simulink model "Adoptive_Cruse_control"  (R2024a)
settings: Solver=FixedStepAuto  StartTime=0.0  StopTime=10.0  RelTol=1e-3
settings Model: DataDictionary=Adoptive_cruse_control_data.sldd  Creator=kanna  LastModifiedBy=kanna
settings OptimizationCC: DefaultParameterBehavior=Inlined  EnhancedBackFolding=on  PassReuseOutputArgsAs=Individual arguments  ZeroExternalMemoryAtStartup=off  ZeroInternalMemoryAtStartup=off  OptimizeBlockOrder=speed  DifferentSizesBufferReuse=on  OptimizationCustomize=off  EfficientTunableParamExpr=on
settings DebuggingCC: ParameterTunabilityLossMsg=error
settings SFSimCC: MATLABDynamicMemAlloc=off
settings RTWCC: Description=Embedded Coder  SystemTargetFile=ert.tlc  TemplateMakefile=ert_default_tmf
settings CodeAppCC: ForceParamTrailComments=on  IgnoreCustomStorageClasses=off  OperatorAnnotations=on  SimulinkDataObjDesc=on  SFDataObjDesc=on  InsertBlockDesc=on
settings ERTTargetCC: TargetLangStandard=C99 (ISO)  GenerateSampleERTMain=on  InlinedParameterPlacement=NonHierarchical  ERTCustomFileTemplate=example_file_process.tlc

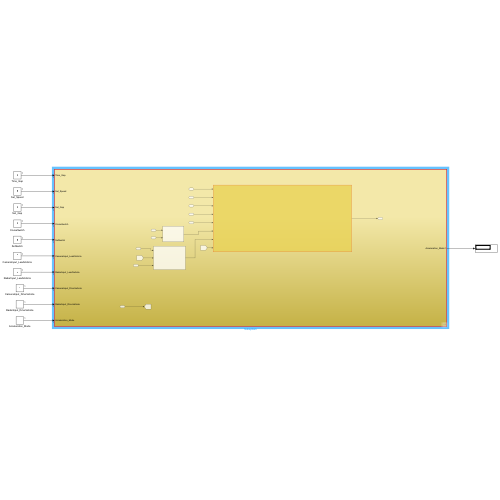
[thumbnail: Simulink's stored preview of the top-level diagram]
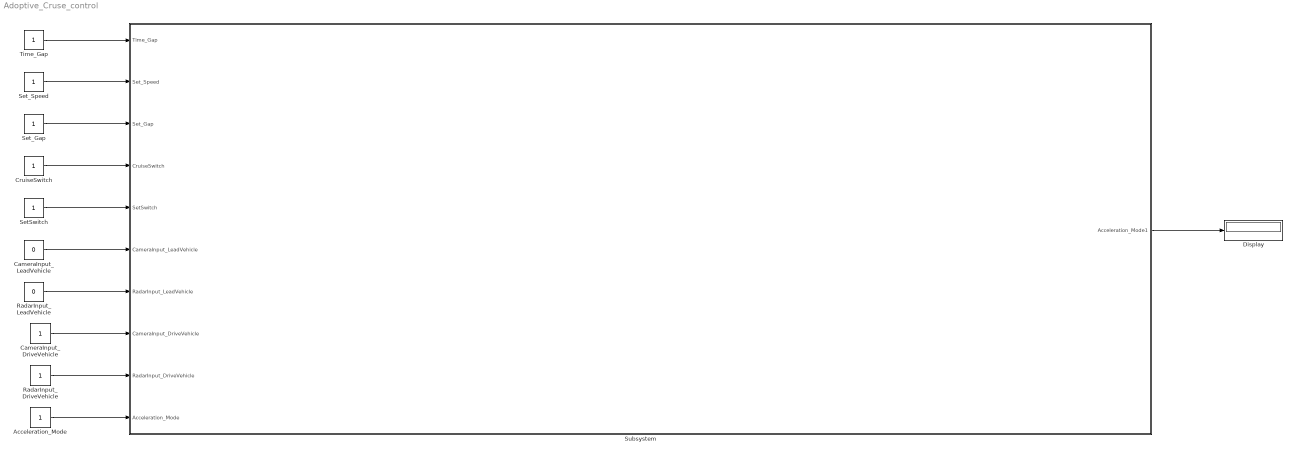
== system Adoptive_Cruse_control ==
  Acceleration_Mode : Constant
  CameraInput_DriveVehicle : Constant
  CameraInput_LeadVehicle : Constant  Value=0
  CruiseSwitch : Constant
  Display : Display
  RadarInput_DriveVehicle : Constant
  RadarInput_LeadVehicle : Constant  Value=0
  SetSwitch : Constant
  Set_Gap : Constant
  Set_Speed : Constant
  Subsystem : Subsystem  TreatAsAtomicUnit=on
  Time_Gap : Constant
  wires:
  Subsystem/1(Acceleration_Mode1) -> Display/1
  Acceleration_Mode/1 -> Subsystem/10(Acceleration_Mode)
  RadarInput_DriveVehicle/1 -> Subsystem/9(RadarInput_DriveVehicle)
  CameraInput_DriveVehicle/1 -> Subsystem/8(CameraInput_DriveVehicle)
  RadarInput_LeadVehicle/1 -> Subsystem/7(RadarInput_LeadVehicle)
  CameraInput_LeadVehicle/1 -> Subsystem/6("CameraInput_LeadVehicle ")
  SetSwitch/1 -> Subsystem/5(SetSwitch)
  CruiseSwitch/1 -> Subsystem/4(CruiseSwitch)
  Set_Gap/1 -> Subsystem/3(Set_Gap)
  Set_Speed/1 -> Subsystem/2(Set_Speed)
  Time_Gap/1 -> Subsystem/1(Time_Gap)

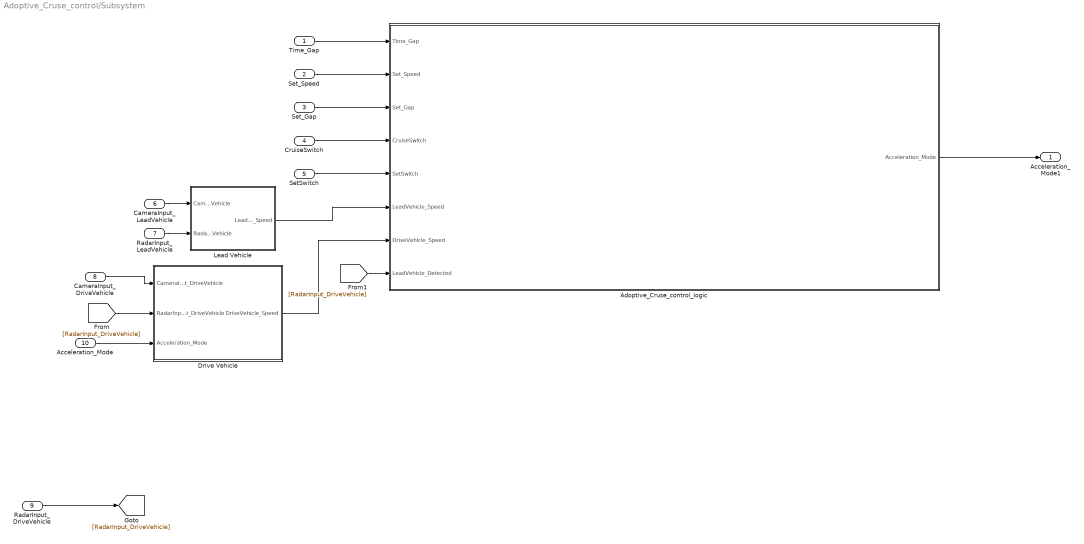
== system Adoptive_Cruse_control/Subsystem ==
  Time_Gap : Inport
  Set_Speed : Inport  Port=2
  Set_Gap : Inport  Port=3
  CruiseSwitch : Inport  Port=4
  SetSwitch : Inport  Port=5
  "CameraInput_LeadVehicle " : Inport  Port=6
  RadarInput_LeadVehicle : Inport  Port=7
  CameraInput_DriveVehicle : Inport  Port=8
  RadarInput_DriveVehicle : Inport  Port=9
  Acceleration_Mode : Inport  Port=10
  Adoptive_Cruse_control_logic : Subsystem
  Drive Vehicle : Subsystem
  Lead Vehicle : Subsystem
  Acceleration_Mode1 : Outport
  wires:
  Drive Vehicle/1("DriveVehicle_Speed ") -> Adoptive_Cruse_control_logic/7("DriveVehicle_Speed ")
  Acceleration_Mode/1 -> Drive Vehicle/3(Acceleration_Mode)
  RadarInput_LeadVehicle/1 -> Lead Vehicle/2(RadarInput_LeadVehicle)
  Set_Gap/1 -> Adoptive_Cruse_control_logic/3(Set_Gap)
  CameraInput_DriveVehicle/1 -> Drive Vehicle/1(CameraInput_DriveVehicle)
  CruiseSwitch/1 -> Adoptive_Cruse_control_logic/4(CruiseSwitch)
  Set_Speed/1 -> Adoptive_Cruse_control_logic/2(Set_Speed)
  Lead Vehicle/1(LeadVehicle_Speed) -> Adoptive_Cruse_control_logic/6(LeadVehicle_Speed)
  "CameraInput_LeadVehicle "/1 -> Lead Vehicle/1("CameraInput_LeadVehicle ")
  SetSwitch/1 -> Adoptive_Cruse_control_logic/5(SetSwitch)
  Time_Gap/1 -> Adoptive_Cruse_control_logic/1(Time_Gap)
  Adoptive_Cruse_control_logic/1(Acceleration_Mode) -> Acceleration_Mode1/1
  RadarInput_DriveVehicle/1 -> [RadarInput_DriveVehicle]
  [RadarInput_DriveVehicle] -> Drive Vehicle/2(RadarInput_DriveVehicle)
  [RadarInput_DriveVehicle] -> Adoptive_Cruse_control_logic/8(LeadVehicle_Detected)

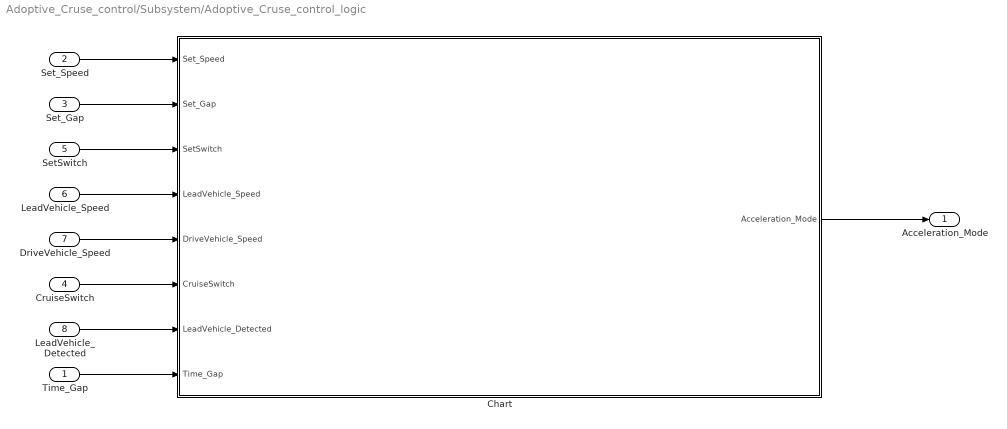
== system Adoptive_Cruse_control/Subsystem/Adoptive_Cruse_control_logic ==
  Time_Gap : Inport
  Set_Speed : Inport  Port=2
  Set_Gap : Inport  Port=3
  CruiseSwitch : Inport  Port=4
  SetSwitch : Inport  Port=5
  LeadVehicle_Speed : Inport  Port=6
  "DriveVehicle_Speed " : Inport  Port=7
  LeadVehicle_Detected : Inport  Port=8
  Chart : Stateflow chart  TreatAsAtomicUnit=on
  Acceleration_Mode : Outport
  wires:
  Time_Gap/1 -> Chart/8(Time_Gap)
  Set_Speed/1 -> Chart/1(Set_Speed)
  Set_Gap/1 -> Chart/2(Set_Gap)
  CruiseSwitch/1 -> Chart/6(CruiseSwitch)
  SetSwitch/1 -> Chart/3(SetSwitch)
  LeadVehicle_Speed/1 -> Chart/4(LeadVehicle_Speed)
  "DriveVehicle_Speed "/1 -> Chart/5("DriveVehicle_Speed ")
  LeadVehicle_Detected/1 -> Chart/7(LeadVehicle_Detected)
  Chart/1(Acceleration_Mode) -> Acceleration_Mode/1

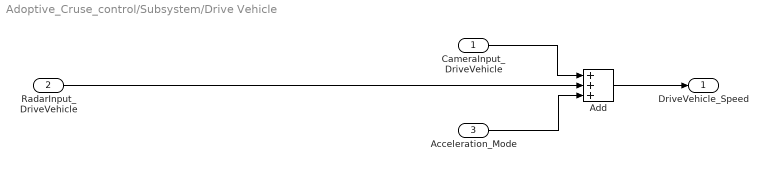
== system Adoptive_Cruse_control/Subsystem/Drive Vehicle ==
  CameraInput_DriveVehicle : Inport
  RadarInput_DriveVehicle : Inport  Port=2
  Acceleration_Mode : Inport  Port=3
  Add : Sum  Inputs=+++
  "DriveVehicle_Speed " : Outport
  wires:
  CameraInput_DriveVehicle/1 -> Add/1
  Add/1 -> "DriveVehicle_Speed "/1
  Acceleration_Mode/1 -> Add/3
  RadarInput_DriveVehicle/1 -> Add/2

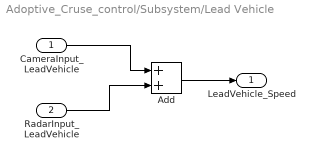
== system Adoptive_Cruse_control/Subsystem/Lead Vehicle ==
  "CameraInput_LeadVehicle " : Inport
  RadarInput_LeadVehicle : Inport  Port=2
  Add : Sum
  LeadVehicle_Speed : Outport
  wires:
  "CameraInput_LeadVehicle "/1 -> Add/1
  Add/1 -> LeadVehicle_Speed/1
  RadarInput_LeadVehicle/1 -> Add/2

== stateflow chart Adoptive_Cruse_control/Subsystem/Adoptive_Cruse_control_logic/Chart ==
  state ACC_OFF_MODE
    en:
    Acceleration_Mode =0
  state ACC_STANDBY_MODE
    en:
    Acceleration_Mode =1
  state ACC_ON_MODE
    en:
    Acceleration_Mode =1
    state LeadVehicle_Not_Detected
      en:
      Acceleration_Mode =1
    state LeadVehicle_Detected_Follow
      en:
      Acceleration_Mode =2
    state LeadVehicle_Speed_lessthan_Set_Speed
      en:
      Acceleration_Mode =4
    state LeadVehicle_Speed_equal_Set_Speed
      en:
      Acceleration_Mode=5
    state LeadVehicle_Not_Detected_Resume
      en:
      Acceleration_Mode =1
    state LeadVehicle_Detected_Resume
      en:
      Acceleration_Mode =3
    (default) -> LeadVehicle_Detected_Follow
    LeadVehicle_Not_Detected -> LeadVehicle_Detected_Follow [order 1] : [[(LeadVehicle_Detected==1) &&...
        |  (DriveVehicle_Speed == Set_Speed) &&...
        |  (LeadVehicle_Speed >= Set_Speed) && ...
        | (Time_Gap >= Set_Gap)]]
    LeadVehicle_Detected_Follow -> LeadVehicle_Not_Detected [order 1] : [(LeadVehicle_Detected == 0)]
    LeadVehicle_Detected_Resume -> LeadVehicle_Detected_Follow [order 1] : [[(DriveVehicle_Speed == Set_Speed) &&...
        |  (LeadVehicle_Speed >= Set_Speed) && ...
        | (Time_Gap >= Set_Gap)]]
    LeadVehicle_Detected_Follow -> LeadVehicle_Speed_lessthan_Set_Speed [order 2] : [(LeadVehicle_Detected == 1) &&...
        |  (LeadVehicle_Speed < Set_Speed) ||...
        |  (Time_Gap < Set_Gap)]
    LeadVehicle_Not_Detected -> LeadVehicle_Speed_lessthan_Set_Speed [order 2] : [[(LeadVehicle_Detected == 1) &&...
        |  (LeadVehicle_Speed < Set_Speed) ||...
        |  (Time_Gap < Set_Gap)]]
    LeadVehicle_Speed_lessthan_Set_Speed -> LeadVehicle_Not_Detected [order 1] : [[(LeadVehicle_Detected == 0) && ...
        | (DriveVehicle_Speed == Set_Speed)]]
    LeadVehicle_Speed_equal_Set_Speed -> LeadVehicle_Speed_lessthan_Set_Speed [order 2] : [[(LeadVehicle_Speed<Set_Speed) && ...
        | (LeadVehicle_Speed<DriveVehicle_Speed) || ...
        | (Time_Gap == 0.75*Set_Gap)]]
    LeadVehicle_Speed_lessthan_Set_Speed -> LeadVehicle_Speed_equal_Set_Speed [order 2] : [[((LeadVehicle_Speed*1.25>=DriveVehicle_Speed) &&...
        |  (LeadVehicle_Speed * 0.75<=DriveVehicle_Speed)) && ...
        | (DriveVehicle_Speed < Set_Speed) && ...
        | ((Time_Gap<=1.25*Set_Gap) && ...
        | (Time_Gap >=0.75*Set_Gap))]]
    LeadVehicle_Speed_equal_Set_Speed -> LeadVehicle_Not_Detected_Resume [order 1] : [[(LeadVehicle_Detected == 0) || ...
        | (DriveVehicle_Speed <= Set_Speed)]]
    LeadVehicle_Speed_equal_Set_Speed -> LeadVehicle_Detected_Resume [order 3] : [[[(DriveVehicle_Speed < Set_Speed) &&...
        |  (LeadVehicle_Speed > DriveVehicle_Speed) ||...
        |  (Time_Gap >= Set_Gap)]]]
    LeadVehicle_Detected_Resume -> LeadVehicle_Speed_equal_Set_Speed [order 3] : [[(DriveVehicle_Speed < Set_Speed) &&...
        |  (LeadVehicle_Speed > DriveVehicle_Speed) && ...
        | (Time_Gap >= Set_Gap)]]
    LeadVehicle_Detected_Resume -> LeadVehicle_Not_Detected_Resume [order 2] : [LeadVehicle_Detected==0]
  (default) -> ACC_OFF_MODE
  ACC_OFF_MODE -> ACC_STANDBY_MODE [order 1] : [CruiseSwitch==1 ]
  ACC_STANDBY_MODE -> ACC_OFF_MODE [order 1] : [CruiseSwitch==0]
  ACC_OFF_MODE -> ACC_ON_MODE [order 2] : [[CruiseSwitch==1&&SetSwitch ==1]]
  ACC_ON_MODE -> ACC_OFF_MODE [order 1] : [CruiseSwitch==0&&SetSwitch ==0]
  ACC_STANDBY_MODE -> ACC_ON_MODE [order 2] : [SetSwitch ==0]
  ACC_ON_MODE -> ACC_STANDBY_MODE [order 2] : [SetSwitch==1]
  data: Set_Speed input; Set_Gap input; SetSwitch input; LeadVehicle_Speed input; DriveVehicle_Speed input; CruiseSwitch input; LeadVehicle_Detected input; Time_Gap input; Acceleration_Mode output
